simulink model "DC_MOTOR_CONTROL_APPLICATION"  (R2021b)
settings: Solver=FixedStepAuto  StartTime=0.0  StopTime=10.0  RelTol=1e-3
PreLoadFcn:
  | clc;
  | clearvars;
  | J = 0.01;
  | b = 0.1;
  | K = 0.01;
  | R = 1;
  | L = 0.5;
  | Ts=0.01;
  | kp=22;
  | ki=41;
  | kd=0.1;
  | up=2000;
settings Model: Creator=sudhir  LastModifiedBy=sudhir

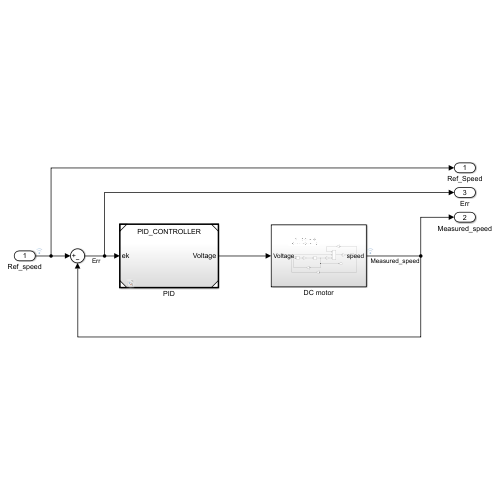
[thumbnail: Simulink's stored preview of the top-level diagram]
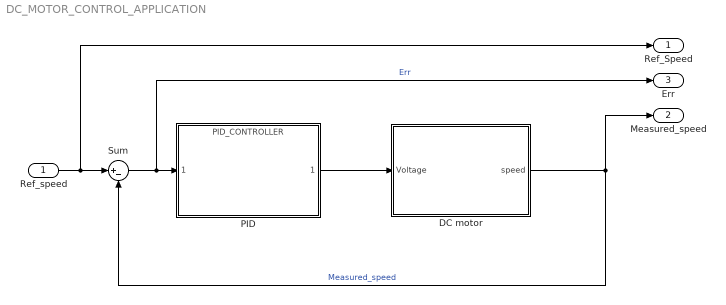
== system DC_MOTOR_CONTROL_APPLICATION ==
  Ref_speed : Inport  OutDataTypeStr=double
  DC motor : Subsystem
  PID : ModelReference  ModelNameDialog=PID_CONTROLLER.slx  SimulationMode=Normal  ModelReferenceVersion=1.42
  Sum : Sum  Inputs=|+-
  Ref_Speed : Outport
  Measured_speed : Outport  Port=2
  Err : Outport  Port=3
  wires:
  Sum/1 -> Err/1, PID/1  "Err"
  DC motor/1(speed) -> Sum/2, Measured_speed/1  "Measured_speed"
  Ref_speed/1 -> Ref_Speed/1, Sum/1
  PID/1 -> DC motor/1(Voltage)

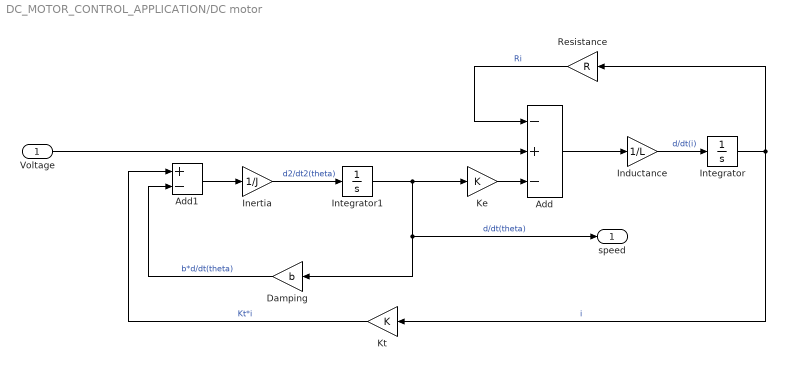
== system DC_MOTOR_CONTROL_APPLICATION/DC motor ==
  Voltage : Inport
  Add : Sum  Inputs=-+-
  Add1 : Sum  Inputs=+-
  Damping : Gain  Gain=b
  Inductance : Gain  Gain=1/L
  Inertia : Gain  Gain=1/J
  Integrator : Integrator
  Integrator1 : Integrator
  Ke : Gain  Gain=K
  Kt : Gain  Gain=K
  Resistance : Gain  Gain=R
  speed : Outport
  wires:
  Voltage/1 -> Add/2
  Inductance/1 -> Integrator/1  "d/dt(i)"
  Ke/1 -> Add/3
  Inertia/1 -> Integrator1/1  "d2/dt2(theta)"
  Resistance/1 -> Add/1  "Ri"
  Damping/1 -> Add1/2  "b*d/dt(theta)"
  Add/1 -> Inductance/1
  Add1/1 -> Inertia/1
  Kt/1 -> Add1/1  "Kt*i"
  Integrator1/1 -> speed/1, Damping/1, Ke/1  "d/dt(theta)"
  Integrator/1 -> Resistance/1, Kt/1  "i"
